simulink model "q3"  (R2018a)
settings: Solver=FixedStepDiscrete  StartTime=0.0  StopTime=0.4  FixedStep=0.000001  RelTol=1e-3
libraries: powerlib x16
settings Model: Creator=MONSTER  LastModifiedBy=MONSTER

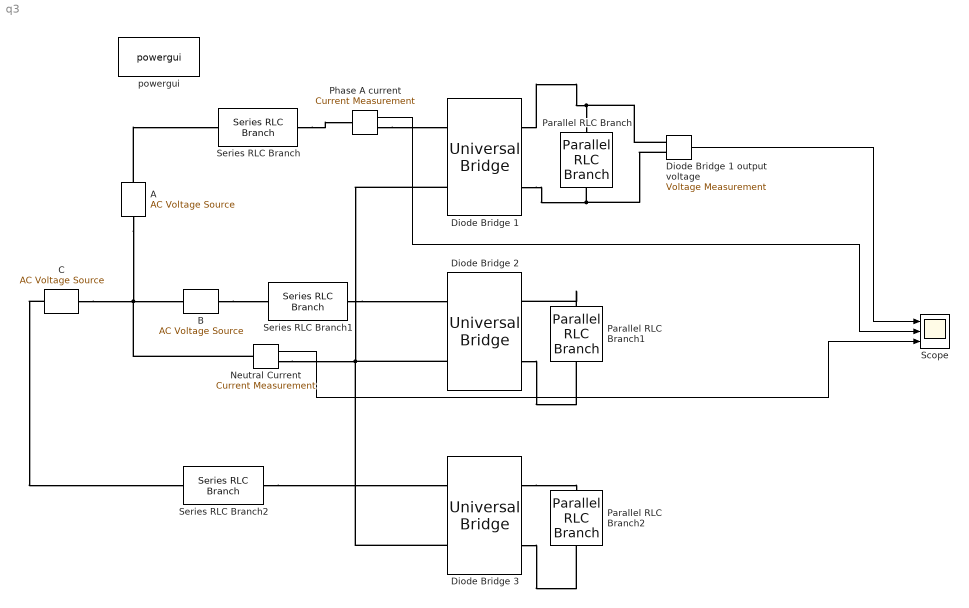
== system q3 ==
  A : powerlib/Electrical Sources/AC Voltage Source  Amplitude=326.6  Phase=0  Frequency=50  SampleTime=0  Measurements=None  BusType=swing  Pref=10e3  Qref=0  Qmin=-inf  Qmax=+inf
  B : powerlib/Electrical Sources/AC Voltage Source  Amplitude=326.6  Phase=120  Frequency=50  SampleTime=0  Measurements=None  BusType=swing  Pref=10e3  Qref=0  Qmin=-inf  Qmax=+inf
  C : powerlib/Electrical Sources/AC Voltage Source  Amplitude=326.6  Phase=240  Frequency=50  SampleTime=0  Measurements=None  BusType=swing  Pref=10e3  Qref=0  Qmin=-inf  Qmax=+inf
  Diode Bridge 1 : powerlib/Power Electronics/Universal Bridge  Arms=2  SnubberResistance=1e5  SnubberCapacitance=inf  Device=Diodes  Ron=1e-3  Lon=0  ForwardVoltages="[  0  0  ]"  ForwardVoltage=0  GTOparameters=[ 10e-6 , 20e-6 ]  IGBTparameters=[ 1e-6 , 2e-6 ]  Measurements=None  Measurements_2=None  converterType=Rectifier
  Diode Bridge 1 output voltage : powerlib/Measurements/Voltage Measurement  PhasorSimulation=off  OutputType=Complex  PSBequivalent=0
  Diode Bridge 2 : powerlib/Power Electronics/Universal Bridge  Arms=2  SnubberResistance=1e5  SnubberCapacitance=inf  Device=Diodes  Ron=1e-3  Lon=0  ForwardVoltages="[  0  0  ]"  ForwardVoltage=0  GTOparameters=[ 10e-6 , 20e-6 ]  IGBTparameters=[ 1e-6 , 2e-6 ]  Measurements=None  Measurements_2=None  converterType=Rectifier
  Diode Bridge 3 : powerlib/Power Electronics/Universal Bridge  Arms=2  SnubberResistance=1e5  SnubberCapacitance=inf  Device=Diodes  Ron=1e-3  Lon=0  ForwardVoltages="[  0  0  ]"  ForwardVoltage=0  GTOparameters=[ 10e-6 , 20e-6 ]  IGBTparameters=[ 1e-6 , 2e-6 ]  Measurements=None  Measurements_2=None  converterType=Rectifier
  Neutral Current : powerlib/Measurements/Current Measurement  PhasorSimulation=off  OutputType=Complex  PSBequivalent=0
  Parallel RLC Branch : powerlib/Elements/Parallel RLC Branch  LConnTagsString=a  RConnTagsString=__new0  BranchType=RC  Resistance=200  Inductance=1e-3  SetiL0=off  InitialCurrent=0  Capacitance=0.00047  Setx0=off  InitialVoltage=0  Measurements=Branch voltage
  Parallel RLC Branch1 : powerlib/Elements/Parallel RLC Branch  LConnTagsString=a  RConnTagsString=__new0  BranchType=RC  Resistance=200  Inductance=1e-3  SetiL0=off  InitialCurrent=0  Capacitance=0.00047  Setx0=off  InitialVoltage=0  Measurements=None
  Parallel RLC Branch2 : powerlib/Elements/Parallel RLC Branch  LConnTagsString=a  RConnTagsString=__new0  BranchType=RC  Resistance=200  Inductance=1e-3  SetiL0=off  InitialCurrent=0  Capacitance=0.00047  Setx0=off  InitialVoltage=0  Measurements=None
  Phase A current : powerlib/Measurements/Current Measurement  PhasorSimulation=off  OutputType=Complex  PSBequivalent=0
  Scope : Scope  NumInputPorts=3
  Series RLC Branch : powerlib/Elements/Series RLC Branch  LConnTagsString=__new0  RConnTagsString=__new0  BranchType=L  Resistance=1  Inductance=0.0006  SetiL0=off  InitialCurrent=0  Capacitance=1e-6  Setx0=off  InitialVoltage=0  Measurements=Branch current
  Series RLC Branch1 : powerlib/Elements/Series RLC Branch  LConnTagsString=__new0  RConnTagsString=__new0  BranchType=L  Resistance=1  Inductance=0.0006  SetiL0=off  InitialCurrent=0  Capacitance=1e-6  Setx0=off  InitialVoltage=0  Measurements=None
  Series RLC Branch2 : powerlib/Elements/Series RLC Branch  LConnTagsString=__new0  RConnTagsString=__new0  BranchType=L  Resistance=1  Inductance=0.0006  SetiL0=off  InitialCurrent=0  Capacitance=1e-6  Setx0=off  InitialVoltage=0  Measurements=None
  powergui : powerlib/powergui  Priority=1  SimulationMode=Discrete  SampleTime=0.000001  frequency=60  Iterations=50  frequencyindice=50  Pbase=100e6  ErrMax=1e-4  UnitsV=kV  UnitsW=MW  buscounter=0  FunctionMessages=off  echomessages=off  EnableUseOfTLC=off  CurrentSourceSwitches=off  DisableSnubberDevices=off  DisableRonSwitches=off  DisableVfSwitches=off  DisplayEquations=off  SolverType=Tustin/Backward Euler (TBE)  Interpol=off  ExternalGateDelay=off  methode=off  Ts=100  x0status=blocks  SPID=off  SwTol=0  HookPort=off  RestoreLinks=warning  ResistiveCurrentMeasurement=off  Frange=[0:2:500]  Ylog=off  Xlog=on  ShowGrid=off  save=off  variable=ZData  structure=input_current  ZoomFFT=off  StartTime=0.05  cycles=10  DisplayStyle=1  fundamental=50  FreqAxis=off  MaxFrequency=1000  frequencyindicesteady=1  RmsSteady=1  display=off
  wires:
  Diode Bridge 1 output voltage/1 -> Scope/1
  Phase A current/1 -> Scope/2
  Neutral Current/1 -> Scope/3
  connections:
  Diode Bridge 2/LConn2 -- Neutral Current/RConn1 -- Diode Bridge 1/LConn2 -- Diode Bridge 3/LConn2
  A/RConn1 -- Series RLC Branch/LConn1
  C/RConn1 -- Series RLC Branch2/LConn1
  B/RConn1 -- Series RLC Branch1/LConn1
  Diode Bridge 1/RConn1 -- Diode Bridge 1 output voltage/LConn1 -- Parallel RLC Branch/LConn1
  Parallel RLC Branch1/LConn1 -- Diode Bridge 2/RConn1
  Diode Bridge 2/RConn2 -- Parallel RLC Branch1/RConn1
  Diode Bridge 3/RConn1 -- Parallel RLC Branch2/LConn1
  Diode Bridge 3/RConn2 -- Parallel RLC Branch2/RConn1
  Series RLC Branch/RConn1 -- Phase A current/LConn1
  Phase A current/RConn1 -- Diode Bridge 1/LConn1
  Diode Bridge 1/RConn2 -- Diode Bridge 1 output voltage/LConn2 -- Parallel RLC Branch/RConn1
  Series RLC Branch2/RConn1 -- Diode Bridge 3/LConn1
  Series RLC Branch1/RConn1 -- Diode Bridge 2/LConn1
  A/LConn1 -- Neutral Current/LConn1 -- B/LConn1 -- C/LConn1
